simulink model "Controller"  (R2022b)
settings: Solver=FixedStepAuto  StartTime=0.0  StopTime=10  FixedStep=0.01  RelTol=1e-3
undefined symbols (not defined in the file or in its folder): params
settings Model: Creator=lulav  LastModifiedBy=lulav
settings DataIOCC: SaveOutput=off  SaveTime=off
settings ModelReferenceCC: ModelReferenceMinAlgLoopOccurrences=on
settings GRTTargetCC: CombineOutputUpdateFcns=off

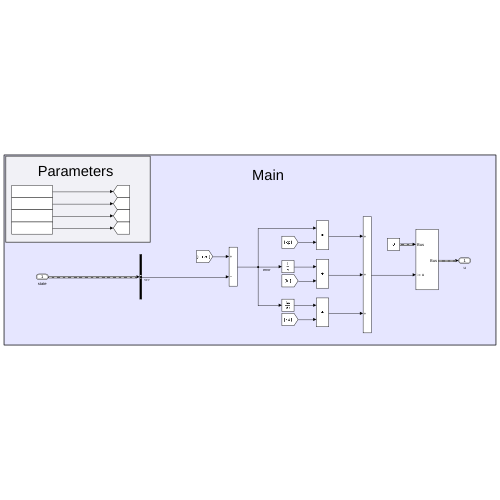
[thumbnail: Simulink's stored preview of the top-level diagram]
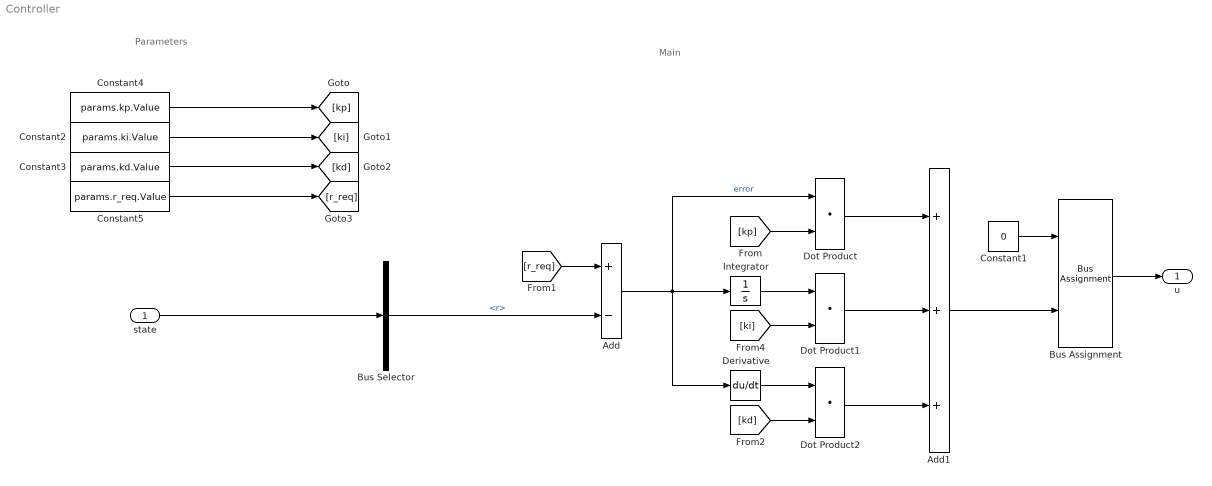
== system Controller ==
  note: Main
  note: Parameters
  state : Inport  OutDataTypeStr=Bus: B_Dynamics  PortDimensions=1  SampleTime=0  BusOutputAsStruct=on
  Add : Sum  Inputs=+-
  Add1 : Sum  Inputs=+++
  Bus Assignment : BusAssignment  AssignedSignals=u
  Bus Selector : BusSelector  OutputSignals=r
  Constant1 : Constant  Value=0  OutDataTypeStr=Bus: B_Controller
  Constant2 : Constant  Value=params.ki.Value
  Constant3 : Constant  Value=params.kd.Value
  Constant4 : Constant  Value=params.kp.Value
  Constant5 : Constant  Value=params.r_req.Value
  Derivative : Derivative
  Dot Product : DotProduct  OutDataTypeStr=Inherit: Inherit via internal rule
  Dot Product1 : DotProduct  OutDataTypeStr=Inherit: Inherit via internal rule
  Dot Product2 : DotProduct  OutDataTypeStr=Inherit: Inherit via internal rule
  Integrator : Integrator
  u : Outport  OutDataTypeStr=Bus: B_Controller  PortDimensions=1  SampleTime=0  BusOutputAsStruct=on
  wires:
  Constant3/1 -> [kd]
  Constant5/1 -> [r_req]
  state/1 -> Bus Selector/1
  Constant2/1 -> [ki]
  Constant4/1 -> [kp]
  Bus Selector/1 -> Add/2  "<r>"
  [r_req] -> Add/1
  Add/1 -> Derivative/1, Dot Product/1, Integrator/1  "error"
  Integrator/1 -> Dot Product1/1
  Derivative/1 -> Dot Product2/1
  [kp] -> Dot Product/2
  [ki] -> Dot Product1/2
  [kd] -> Dot Product2/2
  Dot Product/1 -> Add1/1
  Dot Product1/1 -> Add1/2
  Dot Product2/1 -> Add1/3
  Add1/1 -> Bus Assignment/2
  Bus Assignment/1 -> u/1
  Constant1/1 -> Bus Assignment/1
